simulink model "sin_sampling"  (Simulink 7.2)
settings: Solver=ode3  StartTime=0.0  StopTime=1  RelTol=1e-5
libraries: commutil2 x1, dspbuff3 x1, dspquant2 x1
settings Model: Creator=Administrator  LastModifiedBy=Administrator
settings OptimizationCC: InitFltsAndDblsToZero=on
settings DebuggingCC: MultiTaskCondExecSysMsg=warning

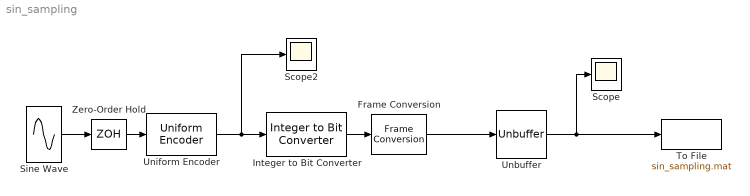
== system sin_sampling ==
  Frame Conversion : FrameConversion
  Integer to Bit Converter : commutil2/Integer to Bit Converter  nbits=8  signedInputValues=Unsigned  bitOrder=MSB first  outDtype=double
  Scope : Scope
  Scope2 : Scope
  Sine Wave : Sin  Frequency=2*pi  SampleTime=0
  To File : ToFile  Filename=sin_sampling.mat  MatrixName=in
  Unbuffer : dspbuff3/Unbuffer  ic=0
  Uniform Encoder : dspquant2/Uniform Encoder  peak=1  bits=8  otype=Unsigned integer
  Zero-Order Hold : ZeroOrderHold  SampleTime=8/504
  wires:
  Sine Wave/1 -> Zero-Order Hold/1
  Zero-Order Hold/1 -> Uniform Encoder/1
  Uniform Encoder/1 -> Integer to Bit Converter/1, Scope2/1
  Integer to Bit Converter/1 -> Frame Conversion/1
  Frame Conversion/1 -> Unbuffer/1
  Unbuffer/1 -> To File/1, Scope/1
